simulink library "INT_EGRVlv_DD"  (R2016b)
settings: Solver=VariableStepAuto  StartTime=0.0  StopTime=10.0  RelTol=1e-3
settings Model: Creator=zhulinfeng  LastModifiedBy=zhulinfeng

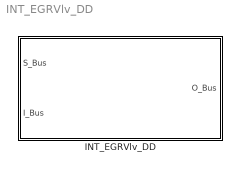
== system INT_EGRVlv_DD ==
  INT_EGRVlv_DD : Subsystem

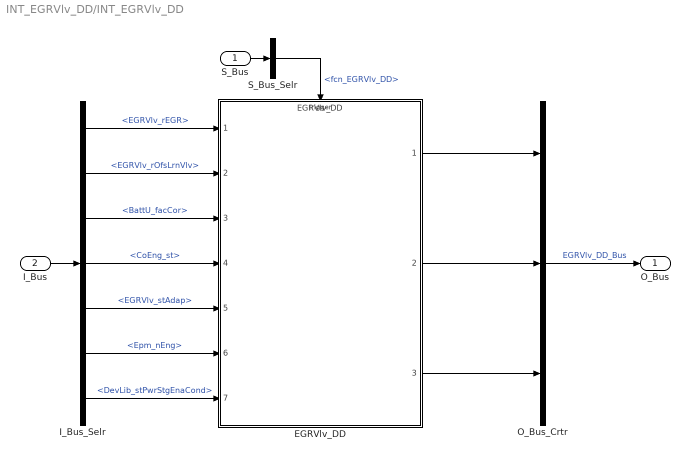
== system INT_EGRVlv_DD/INT_EGRVlv_DD ==
  S_Bus : Inport
  I_Bus : Inport  Port=2
  EGRVlv_DD : ModelReference  ModelNameDialog=EGRVlv_DD  SimulationMode=Normal  ModelReferenceVersion=1.20  TriggerPortName=function  TriggerPortTriggerType=function-call  TriggerPortStatesWhenEnabling=held
  I_Bus_Selr : BusSelector  OutputSignals=EGRVlv_rEGR,EGRVlv_rOfsLrnVlv,BattU_facCor,CoEng_st,EGRVlv_stAdap,Epm_nEng,DevLib_stPwrStgEnaCond
  O_Bus_Crtr : BusCreator  Inputs=3
  S_Bus_Selr : BusSelector  OutputSignals=fcn_EGRVlv_DD
  O_Bus : Outport
  wires:
  S_Bus_Selr/1 -> EGRVlv_DD/Trigger  "<fcn_EGRVlv_DD>"
  S_Bus/1 -> S_Bus_Selr/1
  I_Bus/1 -> I_Bus_Selr/1
  I_Bus_Selr/1 -> EGRVlv_DD/1  "<EGRVlv_rEGR>"
  I_Bus_Selr/2 -> EGRVlv_DD/2  "<EGRVlv_rOfsLrnVlv>"
  I_Bus_Selr/3 -> EGRVlv_DD/3  "<BattU_facCor>"
  I_Bus_Selr/4 -> EGRVlv_DD/4  "<CoEng_st>"
  I_Bus_Selr/5 -> EGRVlv_DD/5  "<EGRVlv_stAdap>"
  I_Bus_Selr/6 -> EGRVlv_DD/6  "<Epm_nEng>"
  I_Bus_Selr/7 -> EGRVlv_DD/7  "<DevLib_stPwrStgEnaCond>"
  O_Bus_Crtr/1 -> O_Bus/1  "EGRVlv_DD_Bus"
  EGRVlv_DD/1 -> O_Bus_Crtr/1
  EGRVlv_DD/2 -> O_Bus_Crtr/2
  EGRVlv_DD/3 -> O_Bus_Crtr/3
